simulink model "DiabetesLC"  (R2023a)
settings: Solver=ode15s  StartTime=0.0  StopTime=10.0  MaxStep=1e-3  RelTol=1e-3
libraries: slpidlib x1
settings Model: Creator=miros  LastModifiedBy=Marco
settings DataIOCC: ReturnWorkspaceOutputs=off  TimeSaveName=t
settings DebuggingCC: AlgebraicLoopMsg=none  ArtificialAlgebraicLoopMsg=none  BlockPriorityViolationMsg=error  MinStepSizeMsg=error  MaxConsecutiveZCsMsg=none  ModelReferenceExtraNoncontSigs=none  OperatingPointInterfaceChecksumMismatchMsg=none

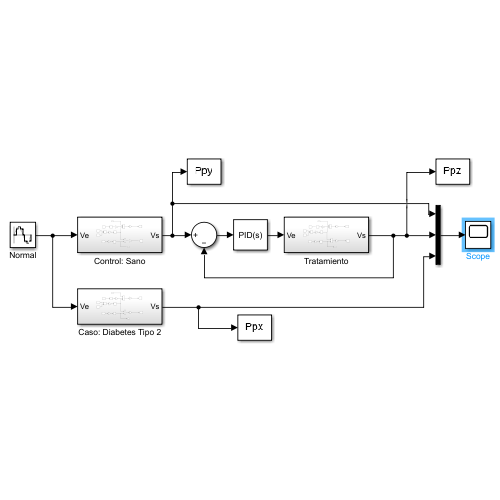
[thumbnail: Simulink's stored preview of the top-level diagram]
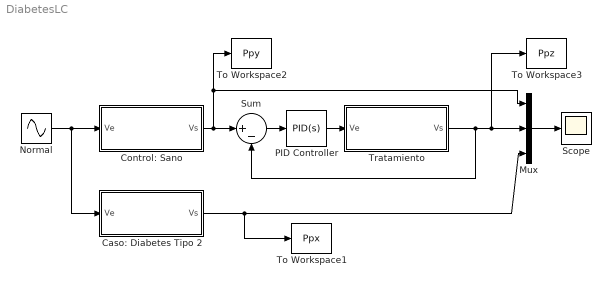
== system DiabetesLC ==
  Caso: Diabetes Tipo 2 : Subsystem
  Control: Sano : Subsystem
  Mux : Mux  Inputs=3
  Normal : Sin  Amplitude=2  Frequency=1.5708  SampleTime=0.001
  PID Controller : slpidlib/PID Controller  Controller=PID  Form=Parallel  TimeDomain=Continuous-time  UseExternalTs=off  SampleTime=-1  IntegratorMethod=Forward Euler  FilterMethod=Forward Euler  ControllerParametersSource=internal  P=209.526932103208  I=4712.72816525048  UseKiTs=off  D=1.13804884347251  N=25472.5950304603  UseFilter=on  TunerSelectOption=Transfer Function Based (PID Tuner App)  InitialConditionSource=internal  InitialConditionForIntegrator=0  InitialConditionForFilter=0  DifferentiatorICPrevScaledInput=0  ExternalReset=none  TrackingMode=off  Kt=1  LimitOutput=off  SatLimitsSource=internal  UpperSaturationLimit=inf  LowerSaturationLimit=-inf  LinearizeAsGain=on  AntiWindupMode=none  Kb=1  LimitIntegrator=off  UpperIntegratorSaturationLimit=inf  LowerIntegratorSaturationLimit=-inf  POutMin=[]  POutMax=[]  IOutMin=[]  IOutMax=[]  DOutMin=[]  DOutMax=[]  NOutMin=[]  NOutMax=[]  SumOutMin=[]  SumOutMax=[]  SaturationOutMin=[]  SaturationOutMax=[]  PParamMin=[]  PParamMax=[]  IParamMin=[]  IParamMax=[]  DParamMin=[]  DParamMax=[]  NParamMin=[]  NParamMax=[]  KbParamMin=[]  KbParamMax=[]  KtParamMin=[]  KtParamMax=[]  KbOutMin=[]  KbOutMax=[]  KtOutMin=[]  KtOutMax=[]  IntegratorOutMin=[]  IntegratorOutMax=[]  FilterOutMin=[]  FilterOutMax=[]  SumI1OutMin=[]  SumI1OutMax=[]  SumI2OutMin=[]  SumI2OutMax=[]  SumI3OutMin=[]  SumI3OutMax=[]  SumI4OutMin=[]  SumI4OutMax=[]  SumDOutMin=[]  SumDOutMax=[]  DifferentiatorOutMin=[]  DifferentiatorOutMax=[]  FilterDiffOutCoefMin=[]  FilterDiffOutCoefMax=[]  ReciprocalOutMin=[]  ReciprocalOutMax=[]  SumDenOutMin=[]  SumDenOutMax=[]  SumNumOutMin=[]  SumNumOutMax=[]  DivideOutMin=[]  DivideOutMax=[]  UdiffTsProdOutMin=[]  UdiffTsProdOutMax=[]  NTsProdOutMin=[]  NTsProdOutMax=[]  UintegralTsProdOutMin=[]  UintegralTsProdOutMax=[]  UngainTsProdOutMin=[]  UngainTsProdOutMax=[]  ClampingZeroOutDataTypeStr=Inherit: Inherit via back propagation  ClampingZeroOutMin=[]  ClampingZeroOutMax=[]  FilterDenConstantOutDataTypeStr=Inherit: Inherit via back propagation  FilterDenConstantOutMin=[]  FilterDenConstantOutMax=[]  PCopyOutDataTypeStr=Inherit: Inherit via back propagation  PCopyOutMin=[]  PCopyOutMax=[]  NCopyOutDataTypeStr=Inherit: Inherit via back propagation  NCopyOutMin=[]  NCopyOutMax=[]  IntegratorContinuousStateAttributes=''  IntegratorStateMustResolveToSignalObject=off  IntegratorRTWStateStorageClass=Auto  FilterContinuousStateAttributes=''  FilterStateMustResolveToSignalObject=off  FilterRTWStateStorageClass=Auto  ParallelPVariant=InternalParameters  IdealPVariant=Disabled  IVariant=InternalParameters  DVariant=InternalParameters  IntegratorVariant=Continuous  SatVariant=Disabled  AWVariant=Passthrough  PCopyVariant=Disabled  TRVariant=Disabled  FdbkBlocksVariant=Forward  IdealPFdbkVariant=Disabled  SatFdbkVariant=Disabled  DerivativeFilterVariant=ContFilter  NVariant=InternalParameters  NCopyVariant=Disabled  FilterICVariant=InternalICsFilter  IntegratorICVariant=InternalICs  ExternalResetVariant=Disabled  TRSumVariant=Passthrough  SumFdbkVariant=Disabled  SumVariant=Sum_PID  TsampFilterVariant=InternalTs  TsampNgainVariant=Passthrough  TsampIntegralVariant=Disabled_SignalSpec  ExternalSaturationOutDataTypeStr=Inherit: Same as second input
  Scope : Scope
  Sum : Sum  Inputs=|+-
  To Workspace1 : ToWorkspace  VariableName=Ppx  SampleTime=-1
  To Workspace2 : ToWorkspace  VariableName=Ppy  SampleTime=-1
  To Workspace3 : ToWorkspace  VariableName=Ppz  SampleTime=-1
  Tratamiento : Subsystem
  wires:
  Mux/1 -> Scope/1
  Control: Sano/1(Vs) -> Sum/1, Mux/1, To Workspace2/1
  PID Controller/1 -> Tratamiento/1(Ve)
  Normal/1 -> Caso: Diabetes Tipo 2/1(Ve), Control: Sano/1(Ve)
  Caso: Diabetes Tipo 2/1(Vs) -> To Workspace1/1, Mux/3
  Sum/1 -> PID Controller/1
  Tratamiento/1(Vs) -> Sum/2, To Workspace3/1, Mux/2

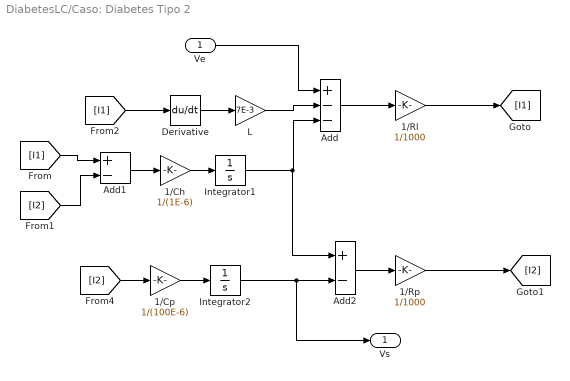
== system DiabetesLC/Caso: Diabetes Tipo 2 ==
  Ve : Inport
  1/Ch : Gain  Gain=1/(1E-6)
  1/Cp : Gain  Gain=1/(100E-6)
  1/Rl : Gain  Gain=1/1000
  1/Rp : Gain  Gain=1/1000
  Add : Sum  Inputs=+--
  Add1 : Sum  Inputs=+-
  Add2 : Sum  Inputs=+-
  Derivative : Derivative
  Integrator1 : Integrator
  Integrator2 : Integrator
  L : Gain  Gain=7E-3
  Vs : Outport
  wires:
  Ve/1 -> Add/1
  Add1/1 -> 1/Ch/1
  [I1] -> Add1/1
  [I2] -> Add1/2
  [I1] -> Derivative/1
  Add/1 -> 1/Rl/1
  1/Rl/1 -> [I1]
  1/Ch/1 -> Integrator1/1
  Integrator1/1 -> Add2/1, Add/3
  Derivative/1 -> L/1
  L/1 -> Add/2
  [I2] -> 1/Cp/1
  1/Cp/1 -> Integrator2/1
  Integrator2/1 -> Vs/1, Add2/2
  Add2/1 -> 1/Rp/1
  1/Rp/1 -> [I2]

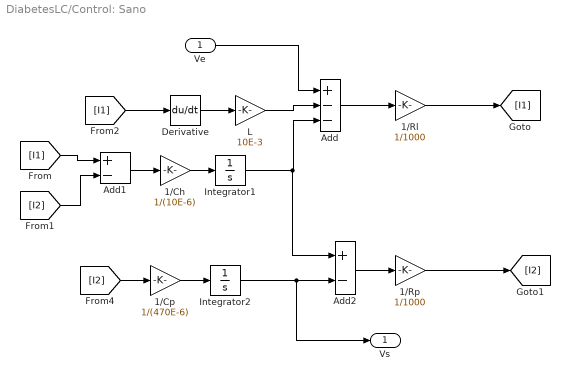
== system DiabetesLC/Control: Sano ==
  Ve : Inport
  1/Ch : Gain  Gain=1/(10E-6)
  1/Cp : Gain  Gain=1/(470E-6)
  1/Rl : Gain  Gain=1/1000
  1/Rp : Gain  Gain=1/1000
  Add : Sum  Inputs=+--
  Add1 : Sum  Inputs=+-
  Add2 : Sum  Inputs=+-
  Derivative : Derivative
  Integrator1 : Integrator
  Integrator2 : Integrator
  L : Gain  Gain=10E-3
  Vs : Outport
  wires:
  Ve/1 -> Add/1
  Add1/1 -> 1/Ch/1
  [I1] -> Add1/1
  [I2] -> Add1/2
  [I1] -> Derivative/1
  Add/1 -> 1/Rl/1
  1/Rl/1 -> [I1]
  1/Ch/1 -> Integrator1/1
  Integrator1/1 -> Add2/1, Add/3
  Derivative/1 -> L/1
  L/1 -> Add/2
  [I2] -> 1/Cp/1
  1/Cp/1 -> Integrator2/1
  Integrator2/1 -> Vs/1, Add2/2
  Add2/1 -> 1/Rp/1
  1/Rp/1 -> [I2]

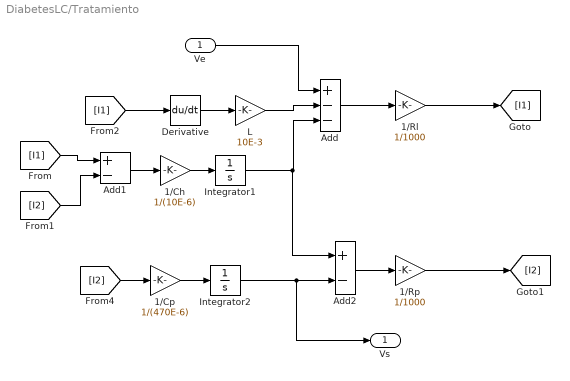
== system DiabetesLC/Tratamiento ==
  Ve : Inport
  1/Ch : Gain  Gain=1/(10E-6)
  1/Cp : Gain  Gain=1/(470E-6)
  1/Rl : Gain  Gain=1/1000
  1/Rp : Gain  Gain=1/1000
  Add : Sum  Inputs=+--
  Add1 : Sum  Inputs=+-
  Add2 : Sum  Inputs=+-
  Derivative : Derivative
  Integrator1 : Integrator
  Integrator2 : Integrator
  L : Gain  Gain=10E-3
  Vs : Outport
  wires:
  Ve/1 -> Add/1
  Add1/1 -> 1/Ch/1
  [I1] -> Add1/1
  [I2] -> Add1/2
  [I1] -> Derivative/1
  Add/1 -> 1/Rl/1
  1/Rl/1 -> [I1]
  1/Ch/1 -> Integrator1/1
  Integrator1/1 -> Add2/1, Add/3
  Derivative/1 -> L/1
  L/1 -> Add/2
  [I2] -> 1/Cp/1
  1/Cp/1 -> Integrator2/1
  Integrator2/1 -> Vs/1, Add2/2
  Add2/1 -> 1/Rp/1
  1/Rp/1 -> [I2]
